simulink model "modelado_simulacion_pendulo"  (R2023a)
settings: Solver=VariableStepAuto  StartTime=0.0  StopTime=2  MaxStep=0.01  RelTol=1e-3
values from neighbouring files (symbols this model uses):
  a1 = 0.2    [practica1.m]
  a2 = 0.1    [practica1.m]
  b1 = 0.3    [practica1.m]
  b2 = 0.25    [practica1.m]
  f = 9.81    [practica1.m]
settings Model: Creator=josel  LastModifiedBy=cash
settings OptimizationCC: ReuseModelBlockBuffer=off

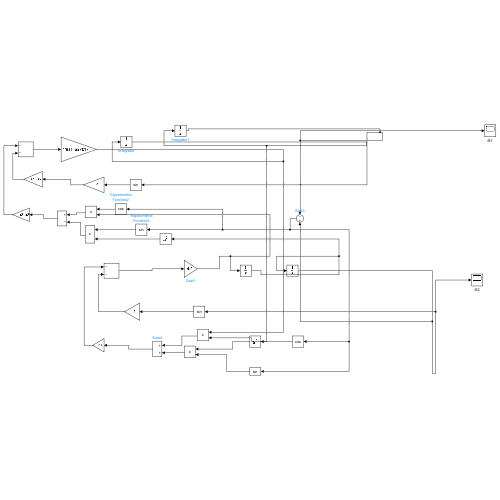
[thumbnail: Simulink's stored preview of the top-level diagram]
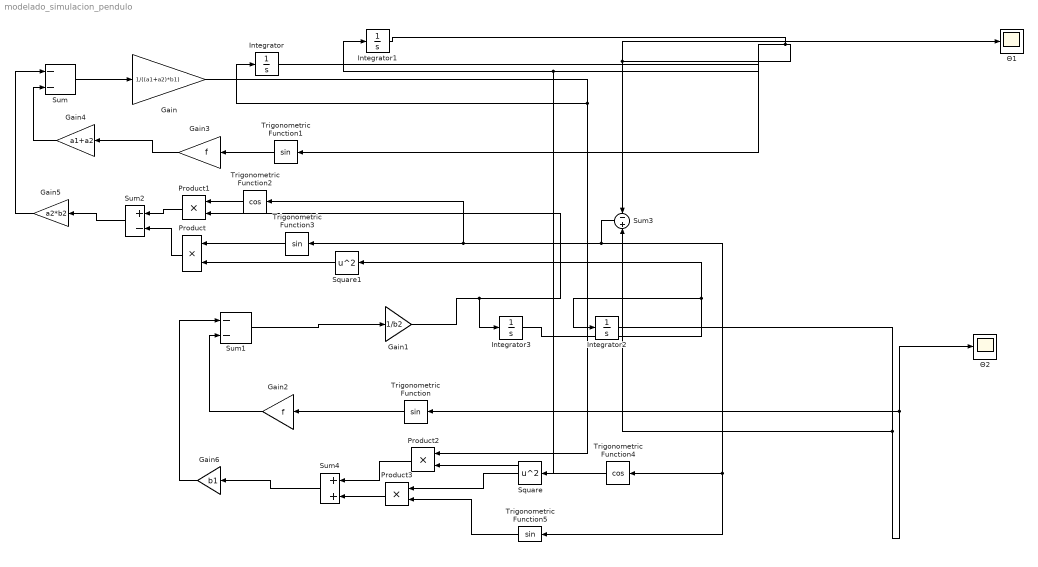
== system modelado_simulacion_pendulo ==
  Gain : Gain  Gain=1/((a1+a2)*b1)
  Gain1 : Gain  Gain=1/b2
  Gain2 : Gain  Gain=f
  Gain3 : Gain  Gain=f
  Gain4 : Gain  Gain=a1+a2
  Gain5 : Gain  Gain=a2*b2
  Gain6 : Gain  Gain=b1
  Integrator : Integrator
  Integrator1 : Integrator
  Integrator2 : Integrator  InitialCondition=(35*pi)/180
  Integrator3 : Integrator
  Product{,1..3} (4 alike) : Product
  Square : Math  Operator=square
  Square1 : Math  Operator=square
  Sum : Sum  Inputs=--
  Sum1 : Sum  Inputs=--
  Sum2 : Sum  Inputs=+-
  Sum3 : Sum  Inputs=-+
  Sum4 : Sum
  Trigonometric Function{,1,3,5} (4 alike) : Trigonometry
  Trigonometric Function2 : Trigonometry  Operator=cos
  Trigonometric Function4 : Trigonometry  Operator=cos
  Θ1 : Scope
  Θ2 : Scope
  wires:
  Gain/1 -> Integrator/1, Product2/1
  Integrator/1 -> Integrator1/1, Square/1
  Gain1/1 -> Product1/2, Integrator3/1
  Integrator3/1 -> Integrator2/1, Square1/1
  Trigonometric Function/1 -> Gain2/1
  Gain2/1 -> Sum1/2
  Sum1/1 -> Gain1/1
  Trigonometric Function1/1 -> Gain3/1
  Gain3/1 -> Gain4/1
  Gain4/1 -> Sum/2
  Sum/1 -> Gain/1
  Gain5/1 -> Sum/1
  Sum2/1 -> Gain5/1
  Product1/1 -> Sum2/1
  Product/1 -> Sum2/2
  Integrator2/1 -> Θ2/1, Trigonometric Function/1, Sum3/2
  Integrator1/1 -> Trigonometric Function1/1, Θ1/1, Sum3/1
  Trigonometric Function2/1 -> Product1/1
  Sum3/1 -> Trigonometric Function5/1, Trigonometric Function4/1, Trigonometric Function3/1, Trigonometric Function2/1
  Square1/1 -> Product/2
  Trigonometric Function3/1 -> Product/1
  Gain6/1 -> Sum1/1
  Sum4/1 -> Gain6/1
  Product2/1 -> Sum4/1
  Product3/1 -> Sum4/2
  Trigonometric Function4/1 -> Product2/2
  Square/1 -> Product3/1
  Trigonometric Function5/1 -> Product3/2
